simulink model "pendulum"  (R2021b)
settings: Solver=FixedStepAuto  StartTime=0.0  StopTime=5  FixedStep=0.01  RelTol=1e-3
model workspace (MAT data in the model file):
  I = 0.016
  M = 1
  g = 10
  l = 0.2
  m = 0.3
settings Model: Creator=DELL  LastModifiedBy=DELL

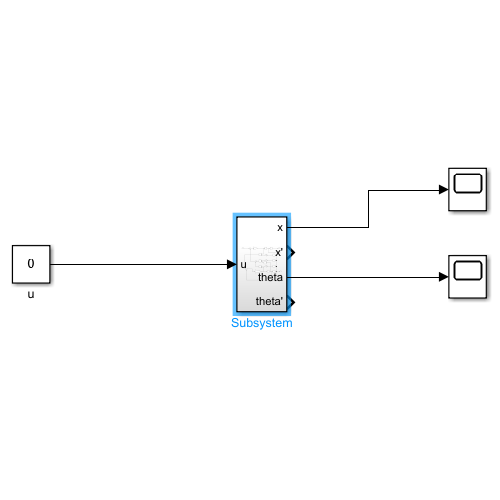
[thumbnail: Simulink's stored preview of the top-level diagram]
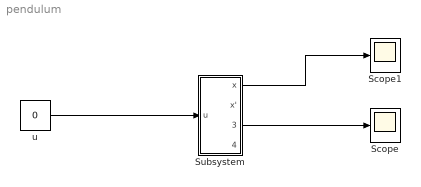
== system pendulum ==
  Scope : Scope
  Scope1 : Scope
  Subsystem : Subsystem
  u : Constant  Value=0
  wires:
  u/1 -> Subsystem/1(u)
  Subsystem/3(theta) -> Scope/1
  Subsystem/1(x) -> Scope1/1

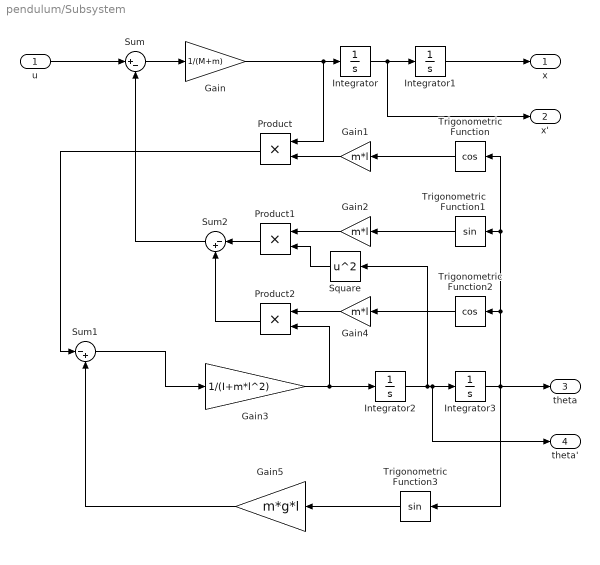
== system pendulum/Subsystem ==
  u : Inport
  Gain : Gain  Gain=1/(M+m)
  Gain1 : Gain  Gain=m*l
  Gain2 : Gain  Gain=m*l
  Gain3 : Gain  Gain=1/(I+m*l^2)
  Gain4 : Gain  Gain=m*l
  Gain5 : Gain  Gain=m*g*l
  Integrator : Integrator
  Integrator1 : Integrator
  Integrator2 : Integrator
  Integrator3 : Integrator  InitialCondition=pi/6
  Product : Product
  Product1 : Product
  Product2 : Product
  Square : Math  Operator=square  SaturateOnIntegerOverflow=on
  Sum : Sum  Inputs=|+-
  Sum1 : Sum  Inputs=|-+
  Sum2 : Sum  Inputs=|-+
  Trigonometric Function : Trigonometry  Operator=cos
  Trigonometric Function1 : Trigonometry
  Trigonometric Function2 : Trigonometry  Operator=cos
  Trigonometric Function3 : Trigonometry
  x : Outport
  x' : Outport  Port=2
  theta : Outport  Port=3
  theta' : Outport  Port=4
  wires:
  Gain5/1 -> Sum1/2
  Gain/1 -> Product/1, Integrator/1
  Square/1 -> Product1/2
  Integrator/1 -> x'/1, Integrator1/1
  Integrator2/1 -> Square/1, theta'/1, Integrator3/1
  Gain4/1 -> Product2/1
  Integrator3/1 -> theta/1, Trigonometric Function3/1, Trigonometric Function/1, Trigonometric Function1/1, Trigonometric Function2/1
  Integrator1/1 -> x/1
  Gain1/1 -> Product/2
  Gain3/1 -> Integrator2/1, Product2/2
  Trigonometric Function/1 -> Gain1/1
  Trigonometric Function2/1 -> Gain4/1
  Product1/1 -> Sum2/1
  Sum/1 -> Gain/1
  u/1 -> Sum/1
  Product2/1 -> Sum2/2
  Product/1 -> Sum1/1
  Sum2/1 -> Sum/2
  Sum1/1 -> Gain3/1
  Gain2/1 -> Product1/1
  Trigonometric Function3/1 -> Gain5/1
  Trigonometric Function1/1 -> Gain2/1
